simulink model "model_4_5_6_tasks"  (R2021b)
settings: Solver=FixedStepAuto  StartTime=0.0  StopTime=10.0  FixedStep=0.001  RelTol=1e-3
undefined symbols (not defined in the file): A1, A2, B1, B2, C2, D2, K1, K2
settings Model: Creator=den  LastModifiedBy=den

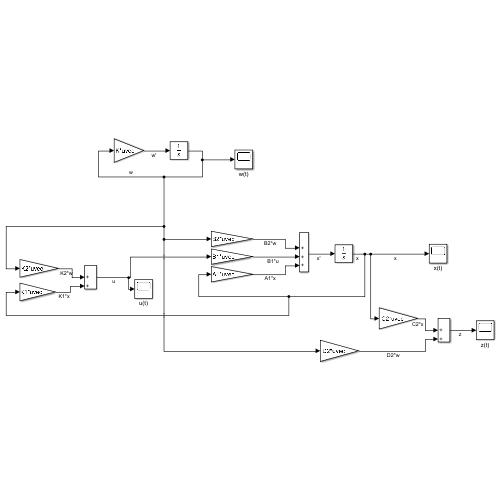
[thumbnail: Simulink's stored preview of the top-level diagram]
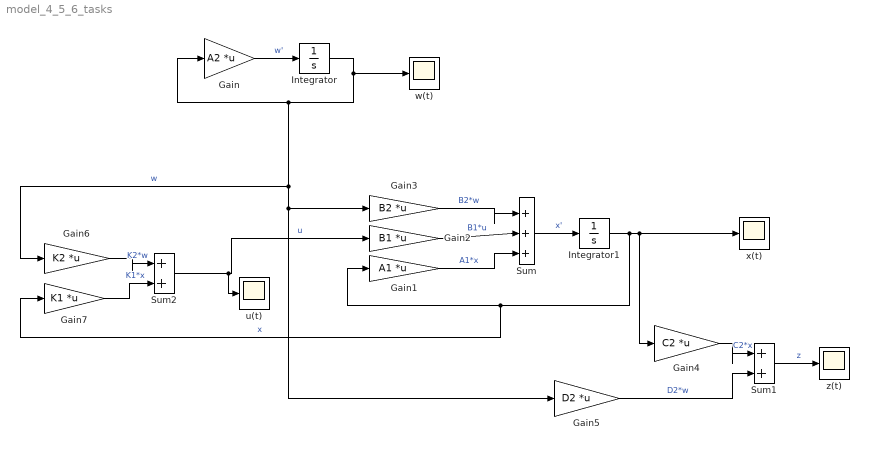
== system model_4_5_6_tasks ==
  Gain : Gain  Gain=A2  Multiplication=Matrix(K*u) (u vector)
  Gain1 : Gain  Gain=A1  Multiplication=Matrix(K*u) (u vector)
  Gain2 : Gain  Gain=B1  Multiplication=Matrix(K*u) (u vector)
  Gain3 : Gain  Gain=B2  Multiplication=Matrix(K*u) (u vector)
  Gain4 : Gain  Gain=C2  Multiplication=Matrix(K*u) (u vector)
  Gain5 : Gain  Gain=D2  Multiplication=Matrix(K*u) (u vector)
  Gain6 : Gain  Gain=K2  Multiplication=Matrix(K*u) (u vector)
  Gain7 : Gain  Gain=K1  Multiplication=Matrix(K*u) (u vector)
  Integrator : Integrator  InitialCondition=[1;1;1;1]
  Integrator1 : Integrator  InitialCondition=[0;0;0]
  Sum : Sum  Inputs=|+++
  Sum1 : Sum  Inputs=|++
  Sum2 : Sum  Inputs=|++
  u(t) : Scope
  w(t) : Scope
  x(t) : Scope
  z(t) : Scope
  wires:
  Gain/1 -> Integrator/1  "w'"
  Integrator/1 -> Gain6/1, Gain5/1, Gain3/1, Gain/1, w(t)/1  "w"
  Sum/1 -> Integrator1/1  "x'"
  Gain3/1 -> Sum/1  "B2*w"
  Gain1/1 -> Sum/3  "A1*x"
  Gain2/1 -> Sum/2  "B1*u"
  Integrator1/1 -> Gain4/1, x(t)/1, Gain7/1, Gain1/1  "x"
  Gain4/1 -> Sum1/1  "C2*x"
  Gain5/1 -> Sum1/2  "D2*w"
  Sum1/1 -> z(t)/1  "z"
  Gain7/1 -> Sum2/2  "K1*x"
  Sum2/1 -> u(t)/1, Gain2/1  "u"
  Gain6/1 -> Sum2/1  "K2*w"
